simulink library "asbAUVlib"  (R2024b)
settings: Solver=VariableStepAuto  StartTime=0.0  StopTime=10.0  RelTol=1e-3
libraries: sharedtransform x3, sharedutil x3
settings Model: Creator=The MathWorks, Inc.  LastModifiedBy=The MathWorks, Inc.
settings OptimizationCC: ReuseModelBlockBuffer=off
settings RTWCC: GPUComputeCapability=3.5

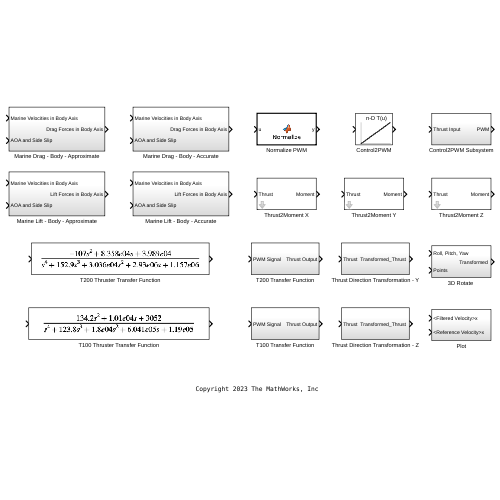
[thumbnail: Simulink's stored preview of the top-level diagram]
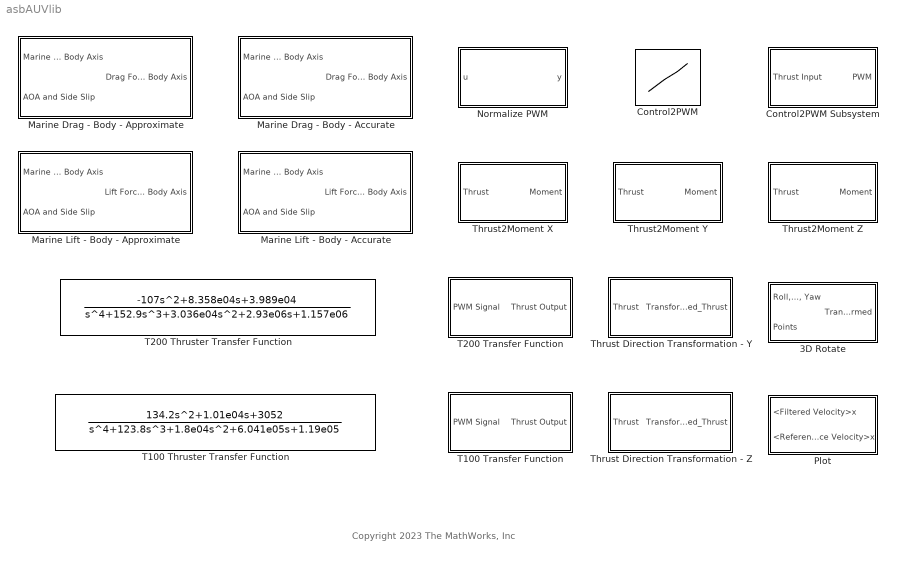
== system asbAUVlib ==
  note: Copyright 2023 The MathWorks, Inc
  "3D Rotate " : Subsystem
  Control2PWM : Lookup_n-D  NumberOfTableDimensions=1  BreakpointsForDimension1=[-1:0.01:1]  Table=1500 + 400 * ([-1:0.01:1])  InternalRulePriority=Speed  RndMeth=Simplest
  Control2PWM Subsystem : Subsystem
  Marine Drag - Body - Accurate : Subsystem
  Marine Drag - Body - Approximate : Subsystem
  Marine Lift - Body - Accurate : Subsystem
  Marine Lift - Body - Approximate : Subsystem
  Normalize PWM : MATLAB Function  TreatAsAtomicUnit=on
  Plot : Subsystem
  T100 Thruster Transfer Function : TransferFcn  Numerator="[134.2 1.01e04  3052]"  Denominator=[1 123.8 1.8e04 6.041e05 1.19e05]
  T100 Transfer Function : Subsystem
  T200 Thruster Transfer Function : TransferFcn  Numerator="[-107  8.358e04  3.989e04]"  Denominator="[1 152.9  3.036e04  2.93e06  1.157e06]"
  T200 Transfer Function : Subsystem
  Thrust Direction Transformation - Y : Subsystem
  Thrust Direction Transformation - Z : Subsystem
  Thrust2Moment X : Subsystem  mask{a=0, b=-0.2, c=0}
      mask prompts: a "X Coordinate of Thruster from Center of Buoyancy"; b "Y Coordinate of Thruster from Center of Buoyancy"; c "Z Coordinate of Thruster from Center of Buoyancy"
      mask DialogControl DescTextVar Prompt: Enter Thruster Position w.r.t Center of Buoyancy
  Thrust2Moment Y : Subsystem  mask{a=.2, b=0, c=0}
      mask prompts: a "X Coordinate of Thruster from Center of Buoyancy"; b "Y Coordinate of Thruster from Center of Buoyancy"; c "Z Coordinate of Thruster from Center of Buoyancy"
      mask DialogControl DescTextVar Prompt: Enter Thruster Position w.r.t Center of Buoyancy
  Thrust2Moment Z : Subsystem  mask{a=0, b=0, c=0}
      mask prompts: a "X Coordinate of Thruster from Center of Buoyancy"; b "Y Coordinate of Thruster from Center of Buoyancy"; c "Z Coordinate of Thruster from Center of Buoyancy"
      mask DialogControl DescTextVar Prompt: Enter Thruster Position w.r.t Center of Buoyancy

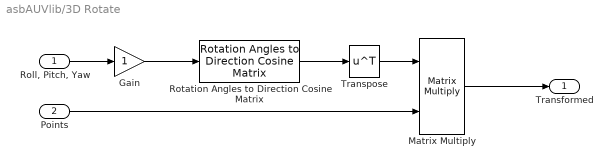
== system asbAUVlib/3D Rotate  ==
  "Roll, Pitch, Yaw" : Inport
  Points : Inport  Port=2
  Gain : Gain
  Matrix Multiply : Product  Multiplication=Matrix(*)
  Rotation Angles to Direction Cosine Matrix : sharedtransform/Rotation Angles to Direction Cosine Matrix  rotationOrder=XYZ  aMode=aMode
  Transpose : Math  Operator=transpose  SignedPower=on
  "Transformed " : Outport  VectorParamsAs1DForOutWhenUnconnected=off
  wires:
  Matrix Multiply/1 -> "Transformed "/1
  Rotation Angles to Direction Cosine Matrix/1 -> Transpose/1
  "Roll, Pitch, Yaw"/1 -> Gain/1
  Transpose/1 -> Matrix Multiply/1
  Gain/1 -> Rotation Angles to Direction Cosine Matrix/1
  Points/1 -> Matrix Multiply/2

== system asbAUVlib/Control2PWM Subsystem ==
  Thrust Input : Inport
  Control2PWM : Lookup_n-D  NumberOfTableDimensions=1  BreakpointsForDimension1=[-1:0.01:1]  Table=1500 + 400 * ([-1:0.01:1])  InternalRulePriority=Speed  RndMeth=Simplest
  PWM : Outport
  wires:
  Thrust Input/1 -> Control2PWM/1
  Control2PWM/1 -> PWM/1

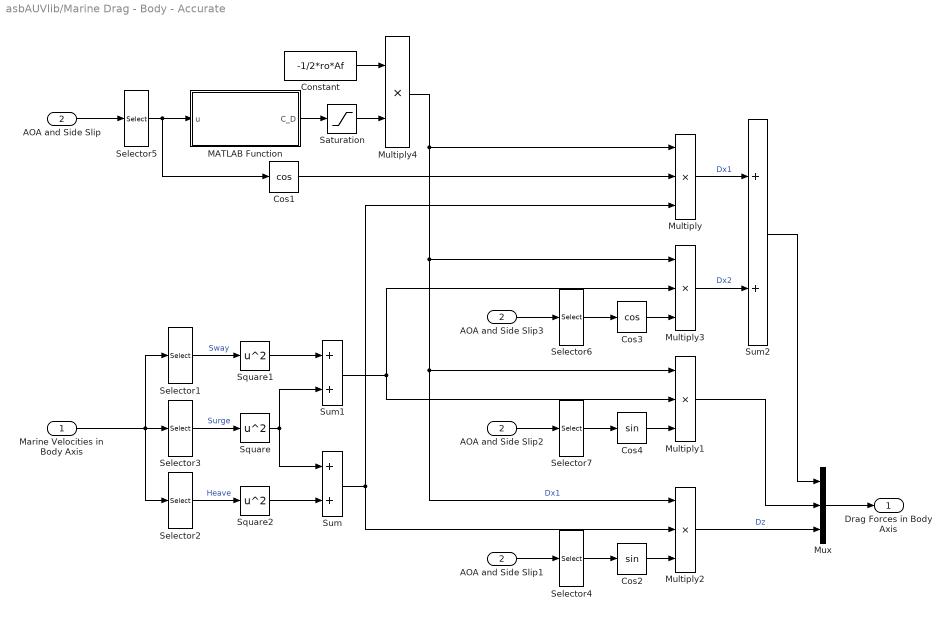
== system asbAUVlib/Marine Drag - Body - Accurate ==
  Marine Velocities in Body Axis : Inport
  AOA and Side Slip : Inport  Port=2
  AOA and Side Slip1 : InportShadow  Port=2
  AOA and Side Slip2 : InportShadow  Port=2
  AOA and Side Slip3 : InportShadow  Port=2
  Constant : Constant  Value=-1/2*ro*Af  mask{ro=1000, Af=0.001}
      mask prompts: ro "Density of Water"; Af "Submarine Frontal Area"
      mask DialogControl DescGroupVar Prompt: Input
      mask DialogControl DescTextVar Prompt: Enter the following values :
  Cos1 : Trigonometry  Operator=cos
  Cos2 : Trigonometry
  Cos3 : Trigonometry  Operator=cos
  Cos4 : Trigonometry
  MATLAB Function : MATLAB Function  TreatAsAtomicUnit=on
  Multiply{,1..3} (4 alike) : Product  Inputs=3
  Multiply4 : Product
  Mux : Mux  Inputs=3
  Saturation : Saturate  UpperLimit=25  LowerLimit=-25
  Selector1 : Selector  InputPortWidth=3  IndexOptions=Index vector (dialog)  Indices=2  OutputSizes=1
  Selector2 : Selector  InputPortWidth=3  IndexOptions=Index vector (dialog)  Indices=3  OutputSizes=1
  Selector{3..5,7} (4 alike) : Selector  InputPortWidth=3  IndexOptions=Index vector (dialog)  Indices=1  OutputSizes=1
  Selector6 : Selector  InputPortWidth=3  IndexOptions=Index vector (dialog)  Indices=2  OutputSizes=1
  Square : Math  Operator=square  SignedPower=on
  Square1 : Math  Operator=square  SignedPower=on
  Square2 : Math  Operator=square  SignedPower=on
  Sum : Sum
  Sum1 : Sum
  Sum2 : Sum
  Drag Forces in Body Axis : Outport  VectorParamsAs1DForOutWhenUnconnected=off
  wires:
  Square1/1 -> Sum1/1
  Multiply1/1 -> Mux/2
  Sum2/1 -> Mux/1
  Cos3/1 -> Multiply3/3
  AOA and Side Slip/1 -> Selector5/1
  Marine Velocities in Body Axis/1 -> Selector1/1, Selector3/1, Selector2/1
  Mux/1 -> Drag Forces in Body Axis/1
  Square2/1 -> Sum/2
  Selector6/1 -> Cos3/1
  Selector5/1 -> Cos1/1, MATLAB Function/1(u)
  MATLAB Function/1(C_D) -> Saturation/1
  Multiply2/1 -> Mux/3  "Dz"
  Cos1/1 -> Multiply/2
  Selector2/1 -> Square2/1  "Heave"
  Multiply3/1 -> Sum2/2  "Dx2"
  Sum/1 -> Multiply/3, Multiply2/2
  Selector3/1 -> Square/1  "Surge"
  Multiply/1 -> Sum2/1  "Dx1"
  Sum1/1 -> Multiply1/2, Multiply3/2
  Cos4/1 -> Multiply1/3
  Selector1/1 -> Square1/1  "Sway"
  Square/1 -> Sum1/2, Sum/1
  Constant/1 -> Multiply4/1
  Saturation/1 -> Multiply4/2
  Multiply4/1 -> Multiply2/1, Multiply1/1, Multiply3/1, Multiply/1  "Dx1"
  AOA and Side Slip1/1 -> Selector4/1
  Selector4/1 -> Cos2/1
  Cos2/1 -> Multiply2/3
  Selector7/1 -> Cos4/1
  AOA and Side Slip2/1 -> Selector7/1
  AOA and Side Slip3/1 -> Selector6/1

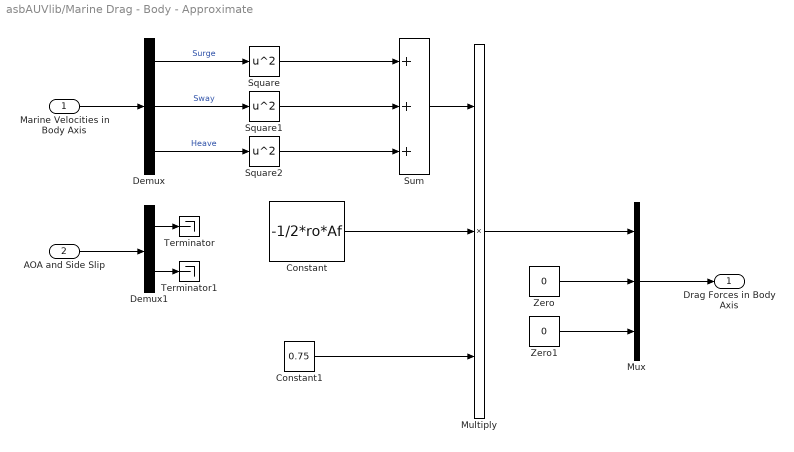
== system asbAUVlib/Marine Drag - Body - Approximate ==
  Marine Velocities in Body Axis : Inport
  AOA and Side Slip : Inport  Port=2
  Constant : Constant  Value=-1/2*ro*Af  mask{ro=1000, Af=0.001}
      mask prompts: ro "Density of Water"; Af "Submarine Frontal Area"
      mask DialogControl DescGroupVar Prompt: Input
      mask DialogControl DescTextVar Prompt: Enter the following values :
  Constant1 : Constant  Value=0.75
  Demux : Demux  Outputs=3
  Demux1 : Demux  Outputs=2
  Multiply : Product  Inputs=3
  Mux : Mux  Inputs=3
  Square : Math  Operator=square  SignedPower=on
  Square1 : Math  Operator=square  SignedPower=on
  Square2 : Math  Operator=square  SignedPower=on
  Sum : Sum  Inputs=+++
  Terminator : Terminator
  Terminator1 : Terminator
  Zero : Constant  Value=0  OutDataTypeStr=Inherit: Inherit via back propagation
  Zero1 : Constant  Value=0  OutDataTypeStr=Inherit: Inherit via back propagation
  Drag Forces in Body Axis : Outport  VectorParamsAs1DForOutWhenUnconnected=off
  wires:
  AOA and Side Slip/1 -> Demux1/1
  Marine Velocities in Body Axis/1 -> Demux/1
  Mux/1 -> Drag Forces in Body Axis/1
  Square2/1 -> Sum/3
  Demux/3 -> Square2/1  "Heave"
  Sum/1 -> Multiply/1
  Demux/1 -> Square/1  "Surge"
  Demux/2 -> Square1/1  "Sway"
  Square/1 -> Sum/1
  Square1/1 -> Sum/2
  Demux1/1 -> Terminator/1
  Demux1/2 -> Terminator1/1
  Constant/1 -> Multiply/2
  Constant1/1 -> Multiply/3
  Multiply/1 -> Mux/1
  Zero/1 -> Mux/2
  Zero1/1 -> Mux/3

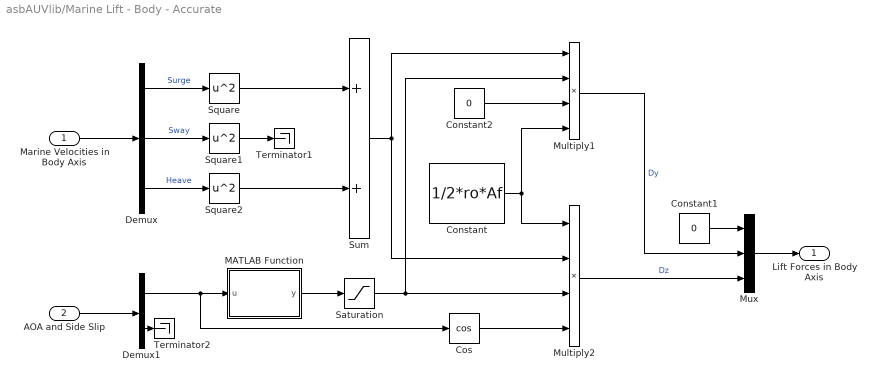
== system asbAUVlib/Marine Lift - Body - Accurate ==
  Marine Velocities in Body Axis : Inport
  AOA and Side Slip : Inport  Port=2
  Constant : Constant  Value=1/2*ro*Af  mask{ro=1000, Af=0.001}
      mask prompts: ro "Density of Water"; Af "Submarine Frontal Area"
      mask DialogControl DescGroupVar Prompt: Input
      mask DialogControl DescTextVar Prompt: Enter the following values :
  Constant1 : Constant  Value=0
  Constant2 : Constant  Value=0
  Cos : Trigonometry  Operator=cos
  Demux : Demux  Outputs=3
  Demux1 : Demux  Outputs=2
  MATLAB Function : MATLAB Function  TreatAsAtomicUnit=on
  Multiply1 : Product  Inputs=4
  Multiply2 : Product  Inputs=4
  Mux : Mux  Inputs=3
  Saturation : Saturate  UpperLimit=25  LowerLimit=-25
  Square : Math  Operator=square  SignedPower=on
  Square1 : Math  Operator=square  SignedPower=on
  Square2 : Math  Operator=square  SignedPower=on
  Sum : Sum
  Terminator1 : Terminator
  Terminator2 : Terminator
  Lift Forces in Body Axis : Outport  VectorParamsAs1DForOutWhenUnconnected=off
  wires:
  Saturation/1 -> Multiply1/2, Multiply2/3
  Constant2/1 -> Multiply1/3
  Multiply2/1 -> Mux/3  "Dz"
  Constant1/1 -> Mux/1
  Cos/1 -> Multiply2/4
  Square/1 -> Sum/1
  Demux/2 -> Square1/1  "Sway"
  Demux/1 -> Square/1  "Surge"
  Sum/1 -> Multiply1/1, Multiply2/2
  Multiply1/1 -> Mux/2  "Dy"
  Demux/3 -> Square2/1  "Heave"
  MATLAB Function/1(y) -> Saturation/1
  Demux1/1 -> MATLAB Function/1(u), Cos/1
  Square2/1 -> Sum/2
  Mux/1 -> Lift Forces in Body Axis/1
  Marine Velocities in Body Axis/1 -> Demux/1
  AOA and Side Slip/1 -> Demux1/1
  Square1/1 -> Terminator1/1
  Demux1/2 -> Terminator2/1
  Constant/1 -> Multiply2/1, Multiply1/4

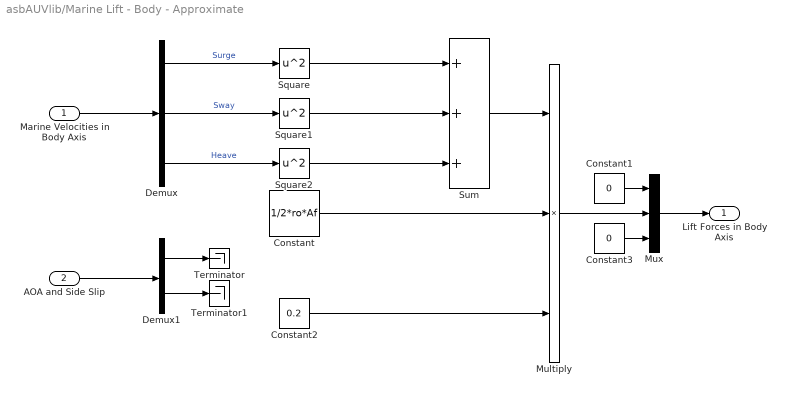
== system asbAUVlib/Marine Lift - Body - Approximate ==
  Marine Velocities in Body Axis : Inport
  AOA and Side Slip : Inport  Port=2
  Constant : Constant  Value=1/2*ro*Af  mask{ro=1000, Af=0.001}
      mask prompts: ro "Density of Water"; Af "Submarine Frontal Area"
      mask DialogControl DescGroupVar Prompt: Input
      mask DialogControl DescTextVar Prompt: Enter the following values :
  Constant1 : Constant  Value=0
  Constant2 : Constant  Value=0.2
  Constant3 : Constant  Value=0
  Demux : Demux  Outputs=3
  Demux1 : Demux  Outputs=2
  Multiply : Product  Inputs=3
  Mux : Mux  Inputs=3
  Square : Math  Operator=square  SignedPower=on
  Square1 : Math  Operator=square  SignedPower=on
  Square2 : Math  Operator=square  SignedPower=on
  Sum : Sum  Inputs=+++
  Terminator : Terminator
  Terminator1 : Terminator
  Lift Forces in Body Axis : Outport  VectorParamsAs1DForOutWhenUnconnected=off
  wires:
  Constant1/1 -> Mux/1
  Square/1 -> Sum/1
  Demux/2 -> Square1/1  "Sway"
  Demux/1 -> Square/1  "Surge"
  Demux/3 -> Square2/1  "Heave"
  Square2/1 -> Sum/3
  Mux/1 -> Lift Forces in Body Axis/1
  Marine Velocities in Body Axis/1 -> Demux/1
  AOA and Side Slip/1 -> Demux1/1
  Square1/1 -> Sum/2
  Sum/1 -> Multiply/1
  Constant/1 -> Multiply/2
  Constant2/1 -> Multiply/3
  Multiply/1 -> Mux/2
  Demux1/1 -> Terminator/1
  Demux1/2 -> Terminator1/1
  Constant3/1 -> Mux/3

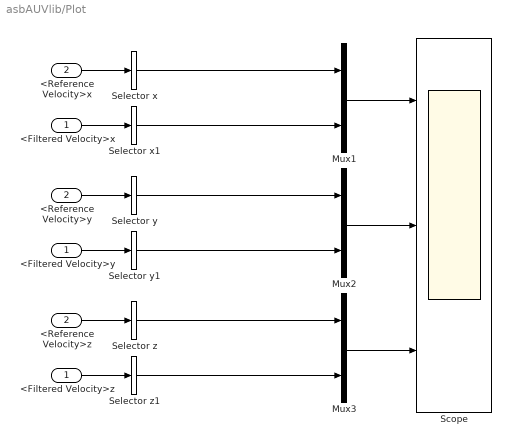
== system asbAUVlib/Plot ==
  <Filtered Velocity>x : Inport
  <Reference Velocity>x : Inport  Port=2
  <Filtered Velocity>y : InportShadow
  <Filtered Velocity>z : InportShadow
  <Reference Velocity>y : InportShadow  Port=2
  <Reference Velocity>z : InportShadow  Port=2
  Mux1 : Mux  Inputs=2
  Mux2 : Mux  Inputs=2
  Mux3 : Mux  Inputs=2
  Scope : Scope  NumInputPorts=3
  Selector x : Selector  InputPortWidth=3  IndexOptions=Index vector (dialog)  Indices=1  OutputSizes=1
  Selector x1 : Selector  InputPortWidth=3  IndexOptions=Index vector (dialog)  Indices=1  OutputSizes=1
  Selector y : Selector  InputPortWidth=3  IndexOptions=Index vector (dialog)  Indices=2  OutputSizes=1
  Selector y1 : Selector  InputPortWidth=3  IndexOptions=Index vector (dialog)  Indices=2  OutputSizes=1
  Selector z : Selector  InputPortWidth=3  IndexOptions=Index vector (dialog)  Indices=2  OutputSizes=1
  Selector z1 : Selector  InputPortWidth=3  IndexOptions=Index vector (dialog)  Indices=2  OutputSizes=1
  wires:
  Mux3/1 -> Scope/3
  Selector x1/1 -> Mux1/2
  Selector y1/1 -> Mux2/2
  Selector z/1 -> Mux3/1
  Mux2/1 -> Scope/2
  Mux1/1 -> Scope/1
  Selector y/1 -> Mux2/1
  Selector x/1 -> Mux1/1
  Selector z1/1 -> Mux3/2
  <Reference Velocity>x/1 -> Selector x/1
  <Reference Velocity>y/1 -> Selector y/1
  <Reference Velocity>z/1 -> Selector z/1
  <Filtered Velocity>x/1 -> Selector x1/1
  <Filtered Velocity>y/1 -> Selector y1/1
  <Filtered Velocity>z/1 -> Selector z1/1

== system asbAUVlib/T100 Transfer Function ==
  PWM Signal : Inport
  T100 Thruster Transfer Function : TransferFcn  Numerator="[134.2 1.01e04  3052]"  Denominator=[1 123.8 1.8e04 6.041e05 1.19e05]
  Thrust Output : Outport
  wires:
  PWM Signal/1 -> T100 Thruster Transfer Function/1
  T100 Thruster Transfer Function/1 -> Thrust Output/1

== system asbAUVlib/T200 Transfer Function ==
  PWM Signal : Inport
  T200 Thruster Transfer Function : TransferFcn  Numerator="[-107  8.358e04  3.989e04]"  Denominator="[1 152.9  3.036e04  2.93e06  1.157e06]"
  Thrust Output : Outport
  wires:
  T200 Thruster Transfer Function/1 -> Thrust Output/1
  PWM Signal/1 -> T200 Thruster Transfer Function/1

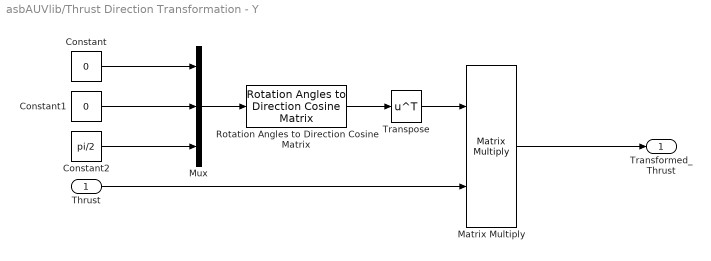
== system asbAUVlib/Thrust Direction Transformation - Y ==
  Thrust : Inport
  Constant : Constant  Value=0
  Constant1 : Constant  Value=0
  Constant2 : Constant  Value=pi/2
  Matrix Multiply : Product  Multiplication=Matrix(*)
  Mux : Mux  Inputs=3
  Rotation Angles to Direction Cosine Matrix : sharedtransform/Rotation Angles to Direction Cosine Matrix  rotationOrder=XYZ  aMode=aMode
  Transpose : Math  Operator=transpose  SignedPower=on
  "Transformed_Thrust " : Outport  VectorParamsAs1DForOutWhenUnconnected=off
  wires:
  Matrix Multiply/1 -> "Transformed_Thrust "/1
  Mux/1 -> Rotation Angles to Direction Cosine Matrix/1
  Rotation Angles to Direction Cosine Matrix/1 -> Transpose/1
  Constant/1 -> Mux/1
  Thrust/1 -> Matrix Multiply/2
  Transpose/1 -> Matrix Multiply/1
  Constant2/1 -> Mux/3
  Constant1/1 -> Mux/2

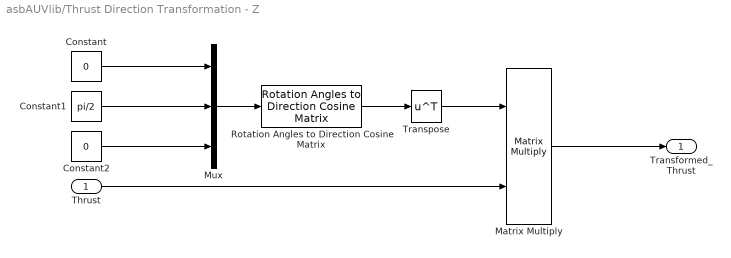
== system asbAUVlib/Thrust Direction Transformation - Z ==
  Thrust : Inport
  Constant : Constant  Value=0
  Constant1 : Constant  Value=pi/2
  Constant2 : Constant  Value=0
  Matrix Multiply : Product  Multiplication=Matrix(*)
  Mux : Mux  Inputs=3
  Rotation Angles to Direction Cosine Matrix : sharedtransform/Rotation Angles to Direction Cosine Matrix  rotationOrder=ZYX  aMode=aMode
  Transpose : Math  Operator=transpose  SignedPower=on
  "Transformed_Thrust " : Outport  VectorParamsAs1DForOutWhenUnconnected=off
  wires:
  Matrix Multiply/1 -> "Transformed_Thrust "/1
  Mux/1 -> Rotation Angles to Direction Cosine Matrix/1
  Rotation Angles to Direction Cosine Matrix/1 -> Transpose/1
  Constant1/1 -> Mux/2
  Thrust/1 -> Matrix Multiply/2
  Constant/1 -> Mux/1
  Transpose/1 -> Matrix Multiply/1
  Constant2/1 -> Mux/3

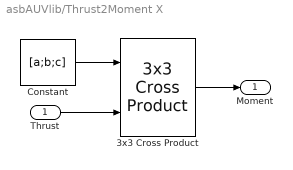
== system asbAUVlib/Thrust2Moment X ==
  Thrust : Inport
  3x3 Cross Product : sharedutil/3x3 Cross Product  aMode=aMode
      settings: LibrarySourceBlock=aerolibutil/3x3 Cross Product
  Constant : Constant  Value=[a;b;c]
  Moment : Outport  VectorParamsAs1DForOutWhenUnconnected=off
  wires:
  3x3 Cross Product/1 -> Moment/1
  Thrust/1 -> 3x3 Cross Product/2
  Constant/1 -> 3x3 Cross Product/1

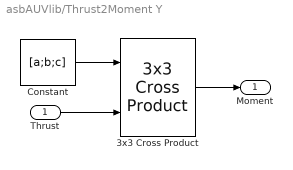
== system asbAUVlib/Thrust2Moment Y ==
  Thrust : Inport
  3x3 Cross Product : sharedutil/3x3 Cross Product  aMode=aMode
      settings: LibrarySourceBlock=aerolibutil/3x3 Cross Product
  Constant : Constant  Value=[a;b;c]
  Moment : Outport  VectorParamsAs1DForOutWhenUnconnected=off
  wires:
  3x3 Cross Product/1 -> Moment/1
  Thrust/1 -> 3x3 Cross Product/2
  Constant/1 -> 3x3 Cross Product/1

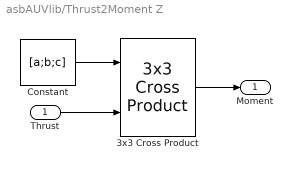
== system asbAUVlib/Thrust2Moment Z ==
  Thrust : Inport
  3x3 Cross Product : sharedutil/3x3 Cross Product  aMode=aMode
      settings: LibrarySourceBlock=aerolibutil/3x3 Cross Product
  Constant : Constant  Value=[a;b;c]
  Moment : Outport  VectorParamsAs1DForOutWhenUnconnected=off
  wires:
  3x3 Cross Product/1 -> Moment/1
  Thrust/1 -> 3x3 Cross Product/2
  Constant/1 -> 3x3 Cross Product/1

== matlab function asbAUVlib/Marine Lift - Body - Accurate/MATLAB Function ==
  data: u input; y output
function y = fcn(u)
if u>pi/2
    u = u-pi;
elseif u < -pi/2
    u = u + pi;
end

y = 1 * (u) + 0;

== matlab function asbAUVlib/Normalize PWM ==
  data: u input; y output
function y = Normalize(u)
y = (u-1500)*150/400;

== matlab function asbAUVlib/Marine Drag - Body - Accurate/MATLAB Function ==
  data: u input; C_D output
function C_D = Calculate_Drag_Coeff(u)
if u>pi/2
    u = u-pi;
elseif u < -pi/2
    u = u + pi;
end
C_D = 5.25*(u.^2) - 0.315 * (u) + 0.732;
